simulink model "sedemo_md1"  (Simulink 7.5)
settings: Solver=VariableStepDiscrete  StartTime=0.0  StopTime=10000  RelTol=1e-3
PostLoadFcn:
  | open_system([gcs '/Arrival Rate Gain']);
undefined symbols (not defined in the file or in its folder): des_figposition
libraries: simulink x4, simeventssink1 x3, simeventsqueue1 x1, simeventsinfo x1, simeventsserver1 x1, simeventsgenerators1 x1
CloseFcn:
  | close_system([gcs '/Arrival Rate Gain']);
settings Model: Creator=The MathWorks Inc.  ExtModeAutoUpdateStatusClock=off
settings DataIOCC: SaveOutput=off  SaveTime=off
settings OptimizationCC: InitFltsAndDblsToZero=on
settings DebuggingCC: SignalResolutionControl=TryResolveAllWithWarning  SolverPrmCheckMsg=none  MultiTaskDSMMsg=warning  MultiTaskCondExecSysMsg=none  StrictBusMsg=Warning
settings RTWCC: IncludeERTFirstTime=on
settings SimEventsCC: propDiagAttribOutput=1  propDiagFcnCallOutput=1  propDiagStatOutput=0

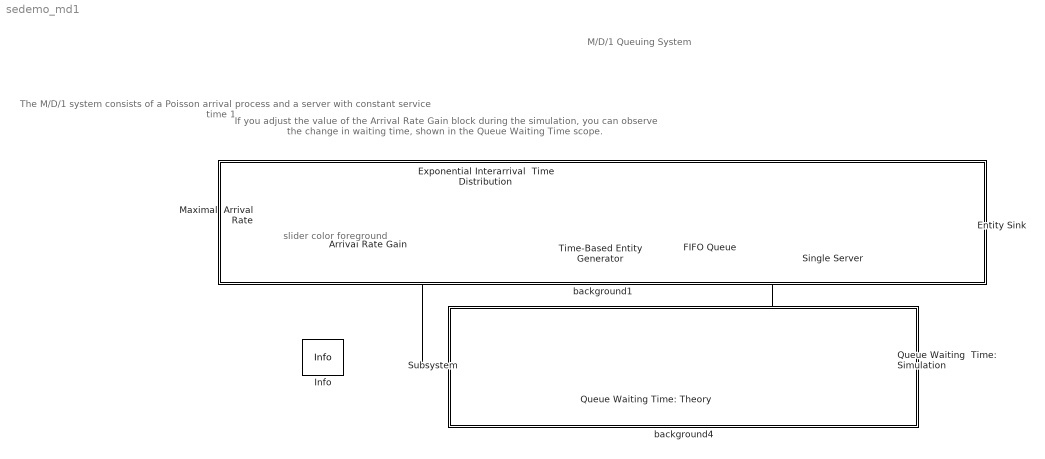
== system sedemo_md1 ==
  note: The M/D/1 system consists of a
      | Poisson arrival process and a
      | server with constant service time 1.
  note: M/D/1 Queuing System
  note: slider color foreground
  note: If you adjust the value of the Arrival Rate
      | Gain block during the simulation, you
      | can observe the change in waiting time,
      | shown in the Queue Waiting Time scope.
  Arrival Rate Gain : simulink/Math Operations/Slider Gain  SystemSampleTime=-1  low=0.1  gain=0.4  high=0.999
  Entity Sink : simeventssink1/Entity Sink  Priority=1  SystemSampleTime=-1  AvailableForArrivals=on  StatNumberArrived=Off
  Exponential Interarrival  Time Distribution : Subsystem  mask(Exponential Random Number Generator){seed=60790}
      mask prompts: seed "Initial seed"
      mask help: Output exponentially distributed random numbers with the input rate. Output is repeatable for a given seed.
      mask Display: disp('Exponential\nGeneration');
  FIFO Queue : simeventsqueue1/FIFO Queue  Priority=1  SystemSampleTime=-1  Capacity=Inf  EnableTOPort=off  StatNumberDeparted=Off  StatNumberInBlock=Off  StatPendingEntity=Off  StatAverageWait=On  StatAverageQueueLength=Off  StatNumberTimedout=Off
  Info : simeventsinfo/Info  SystemSampleTime=-1
  Maximal  Arrival Rate : Constant  OutDataType=sfix(16)  OutScaling=2^0
  Queue Waiting Time: Theory : simeventssink1/Signal Scope  Priority=1  SystemSampleTime=-1  PlotType=Stair  InputType=Signal  NumInputs=1  AttributeNameY=Count  XInputOptionSignal=Event time  XInputOptionEntity=Event time  AttributeNameX=Count  EnableEntityOutport=on  XMin=0  XMax=10  XLimitExceededOption=Stretch axis limits  YLimitExceededOption=Stretch axis limits  AxisGrid=on  AxisLegend=off  LineDisables=""  LineColors=b  LineStyles=-  LineMarkers=.  OpenScopeAtSimStart=on  Title=Queue Waiting Time : Theory  YLabel=Waiting Time  XLabel=Time  FigurePosition=des_figposition([5 10 25 25])  AxisZoom=off  DataStoreOption=Limited  DataPointsLimit=10000  StatNumberArrived=Off  ShowCountPlotted=off  ShowToolbar=on
      settings: YMin=0  YMax=1
  Queue Waiting  Time: Simulation : simeventssink1/Signal Scope  Priority=1  SystemSampleTime=-1  PlotType=Stair  InputType=Signal  NumInputs=1  AttributeNameY=Count  XInputOptionSignal=Event time  XInputOptionEntity=Event time  AttributeNameX=Count  EnableEntityOutport=on  XMin=0  XMax=10  XLimitExceededOption=Stretch axis limits  YLimitExceededOption=Stretch axis limits  AxisGrid=on  AxisLegend=off  LineDisables=""  LineColors=b  LineStyles=-  LineMarkers=.  OpenScopeAtSimStart=on  Title=Queue Waiting Time : Simulation  YLabel=Waiting Time  XLabel=Time  FigurePosition=des_figposition([33 10 25 25])  AxisZoom=off  DataStoreOption=Limited  DataPointsLimit=10000  StatNumberArrived=Off  ShowCountPlotted=off  ShowToolbar=on
      settings: YMin=0  YMax=2
  Single Server : simeventsserver1/Single Server  Priority=1  SystemSampleTime=-1  ServiceTimeFrom=Dialog  ServiceTime=1  AttributeName=ServiceTime  PriorityServiceCompletion=500  PermitPreemption=off  SortingAttributeName=PriorityAttributeName  SortingDirection=Ascending  WriteToAttribute=off  ResidualAttributeName=ResidualServiceTime  CreateAttribute=on  EnableTOPort=off  StatNumberDeparted=Off  StatNumberInBlock=Off  StatNumberPreempted=Off  StatPendingEntity=Off  StatAverageWait=Off  StatUtilization=Off  StatNumberTimedout=Off
      settings: AttributesFormatString=Service Time = %<ServiceTime>
  Subsystem : Subsystem
      mask Type: M/D/1 Waiting Time Evaluation
      mask Description: Evaluate M/D/1 waiting time for the input arrival rate and service rate=1. Combine it with simulation result and output.
      mask Display: disp('Waiting Time\nEvaluation');
  Time-Based Entity Generator : simeventsgenerators1/Entity Generators/Time-Based Entity Generator  Priority=1  DialogController=des_ddg_create  DialogControllerArgs=DataTag6  SystemSampleTime=-1  GenerateEntitiesUpon=Intergeneration time from port t  Distribution=Constant  Minimum=0  Maximum=1  Mean=1  InitialSeed=12345  Period=1  PriorityEntityGeneration=1  GenerateEntityAtSimulationStart=on  ResponseWhenBlocked=Error  ResponseWhenUnblocked=Immediate restart  EntityType=Standard  StatNumberDeparted=Off  StatPendingEntity=Off  StatAverageIntergenerationTime=Off
  background1 : Subsystem
      mask Display: disp('')
  background4 : Subsystem
      mask Display: disp('')
  wires:
  Maximal  Arrival Rate/1 -> Arrival Rate Gain/1
  Exponential Interarrival  Time Distribution/1(Out1) -> Time-Based Entity Generator/1
  Arrival Rate Gain/1 -> Exponential Interarrival  Time Distribution/1(rate), Subsystem/1(lambda)
  Subsystem/1(Out1) -> Queue Waiting Time: Theory/1
  FIFO Queue/1 -> Queue Waiting  Time: Simulation/1
  connections:
  FIFO Queue/RConn1 -- Single Server/LConn1
  Single Server/RConn1 -- Entity Sink/LConn1
  Time-Based Entity Generator/RConn1 -- FIFO Queue/LConn1

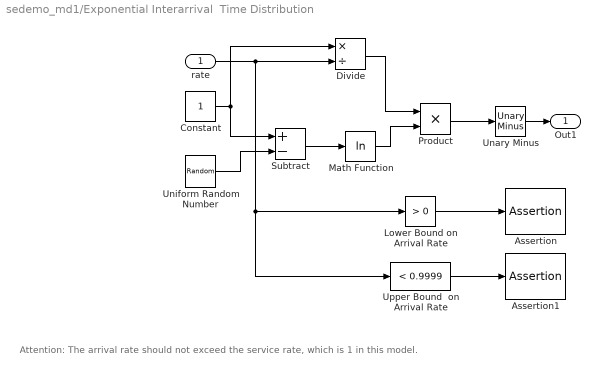
== system sedemo_md1/Exponential Interarrival  Time Distribution ==
  note: Attention: The arrival rate
      | should not exceed the service
      | rate, which is 1 in this model.
  rate : Inport  OutDataType=sfix(16)  OutScaling=2^0
  Assertion : Assertion  Enabled=on
  Assertion1 : Assertion  Enabled=on
  Constant : Constant  OutDataType=sfix(16)  OutScaling=2^0
  Divide : Product  Inputs=*/  OutDataType=sfix(16)  OutScaling=2^-10
  Lower Bound on Arrival Rate : simulink/Logic and Bit Operations/Compare To Constant  SystemSampleTime=-1  relop=>  const=0  LogicOutDataTypeMode=uint8  ZeroCross=off
  Math Function : Math  Operator=log  OutDataType=sfix(16)  OutScaling=2^0  SaturateOnIntegerOverflow=on
  Product : Product  OutDataType=sfix(16)  OutScaling=2^0  RndMeth=Zero
  Subtract : Sum  Inputs=+-  OutDataType=sfix(16)  OutScaling=2^-10
  Unary Minus : simulink/Math Operations/Unary Minus  DoSatur=off
  Uniform Random Number : UniformRandomNumber  Minimum=0  Seed=seed  SampleTime=0
  "Upper Bound  on Arrival Rate " : simulink/Logic and Bit Operations/Compare To Constant  SystemSampleTime=-1  relop=<  const=0.9999  LogicOutDataTypeMode=uint8  ZeroCross=off
  Out1 : Outport  OutDataType=sfix(16)  OutScaling=2^0
  wires:
  "Upper Bound  on Arrival Rate "/1 -> Assertion1/1
  Lower Bound on Arrival Rate/1 -> Assertion/1
  Divide/1 -> Product/1
  rate/1 -> "Upper Bound  on Arrival Rate "/1, Lower Bound on Arrival Rate/1, Divide/2
  Constant/1 -> Divide/1, Subtract/1
  Uniform Random Number/1 -> Subtract/2
  Subtract/1 -> Math Function/1
  Math Function/1 -> Product/2
  Product/1 -> Unary Minus/1
  Unary Minus/1 -> Out1/1

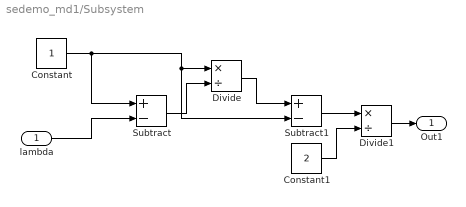
== system sedemo_md1/Subsystem ==
  lambda : Inport  OutDataType=sfix(16)  OutScaling=2^0
  Constant : Constant  OutDataType=sfix(16)  OutScaling=2^0
  Constant1 : Constant  Value=2  OutDataType=sfix(16)  OutScaling=2^0
  Divide : Product  Inputs=*/  OutDataType=sfix(16)  OutScaling=2^-10
  Divide1 : Product  Inputs=*/  OutDataType=sfix(16)  OutScaling=2^-10
  Subtract : Sum  Inputs=+-  OutDataType=sfix(16)  OutScaling=2^-10
  Subtract1 : Sum  Inputs=+-  OutDataType=sfix(16)  OutScaling=2^-10
  Out1 : Outport  OutDataType=sfix(16)  OutScaling=2^0
  wires:
  Constant1/1 -> Divide1/2
  Subtract1/1 -> Divide1/1
  Divide/1 -> Subtract1/1
  Subtract/1 -> Divide/2
  Constant/1 -> Subtract/1, Subtract1/2, Divide/1
  lambda/1 -> Subtract/2
  Divide1/1 -> Out1/1

== system sedemo_md1/background1 ==

== system sedemo_md1/background4 ==
